simulink model "Khajuriwala_rishi_rbe_595_hw_08_simulink"  (R2017b)
settings: Solver=VariableStepAuto  StartTime=0.0  StopTime=10  RelTol=1e-3
values from neighbouring files (symbols this model uses):
  bc = bh    (= 25)    [Khajuriwala_rishi_rbe_595_hw_08_initialization_file.m]
  bh = 25    [Khajuriwala_rishi_rbe_595_hw_08_initialization_file.m]
  Bt = 300    [Khajuriwala_rishi_rbe_595_hw_08_initialization_file.m]    (also in virtualcoupling3.m = block.DialogPrm(2).Data)
  Bvc = 3    [Khajuriwala_rishi_rbe_595_hw_08_initialization_file.m]    (also in virtualcoupling1.m = block.DialogPrm(2).Data)
  Fh = 5    [Khajuriwala_rishi_rbe_595_hw_08_initialization_file.m]
  fh1 = 5    [Khajuriwala_rishi_rbe_595_hw_08_initialization_file.m]
  Kt = 2000    [Khajuriwala_rishi_rbe_595_hw_08_initialization_file.m]    (also in virtualcoupling3.m = block.DialogPrm(1).Data)
  Kvc = 2000    [Khajuriwala_rishi_rbe_595_hw_08_initialization_file.m]    (also in virtualcoupling1.m = block.DialogPrm(1).Data)
  mc = 20    [Khajuriwala_rishi_rbe_595_hw_08_initialization_file.m]
  mh = 10    [Khajuriwala_rishi_rbe_595_hw_08_initialization_file.m]
  vc0 = vhd0    (= 0)    [Khajuriwala_rishi_rbe_595_hw_08_initialization_file.m]
  vhd0 = 0    [Khajuriwala_rishi_rbe_595_hw_08_initialization_file.m]
  xc0 = xhd0    (= -0.05)    [Khajuriwala_rishi_rbe_595_hw_08_initialization_file.m]
  xhd0 = -0.05    [Khajuriwala_rishi_rbe_595_hw_08_initialization_file.m]
settings Model: Creator=Lhotse  LastModifiedBy=Lhotse

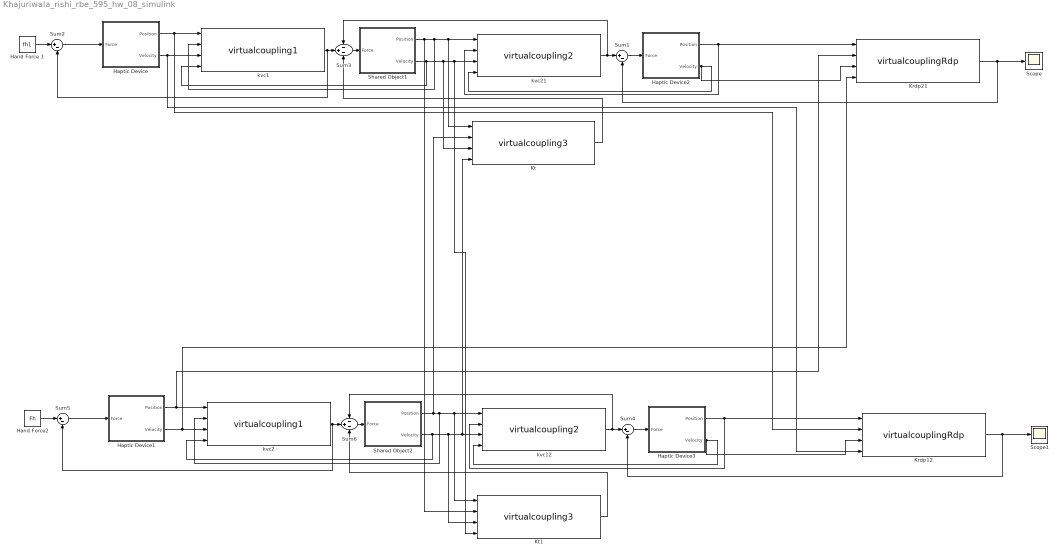
== system Khajuriwala_rishi_rbe_595_hw_08_simulink ==
  Hand Force 1 : Constant  Value=fh1
  Hand Force2 : Constant  Value=Fh
  Haptic Device : Subsystem
  Haptic Device1 : Subsystem
  Haptic Device2 : Subsystem
  Haptic Device3 : Subsystem
  Krdp12 : M-S-Function  FunctionName=virtualcouplingRdp  Parameters=Krdp, Brdp
  Krdp21 : M-S-Function  FunctionName=virtualcouplingRdp  Parameters=Krdp, Brdp
  Kt : M-S-Function  FunctionName=virtualcoupling3  Parameters=Kt,Bt
  Kt1 : M-S-Function  FunctionName=virtualcoupling3  Parameters=Kt,Bt
  Scope : Scope
  Scope1 : Scope
  Shared Object1 : Subsystem
  Shared Object2 : Subsystem
  Sum{1..2,4..5} (4 alike) : Sum  Inputs=|+-
  Sum3 : Sum  Inputs=-+-
  Sum6 : Sum  Inputs=-+-
  kvc1 : M-S-Function  FunctionName=virtualcoupling1  Parameters=Kvc,Bvc
  kvc12 : M-S-Function  FunctionName=virtualcoupling2  Parameters=Kvc,Bvc
  kvc2 : M-S-Function  FunctionName=virtualcoupling1  Parameters=Kvc,Bvc
  kvc21 : M-S-Function  FunctionName=virtualcoupling2  Parameters=Kvc,Bvc
  wires:
  Haptic Device/1(Position) -> Krdp12/2, kvc1/1
  Shared Object1/2(Velocity) -> Kt/3, Kt1/4, kvc21/3, kvc1/4
  Haptic Device2/2(Velocity) -> kvc21/4, Krdp21/3
  Haptic Device/2(Velocity) -> Krdp12/4, kvc1/3
  Shared Object1/1(Position) -> Kt1/2, Kt/1, kvc21/1, kvc1/2
  Sum2/1 -> Haptic Device/1(Force)
  Haptic Device2/1(Position) -> kvc21/2, Krdp21/1
  Hand Force 1/1 -> Sum2/1
  kvc21/1 -> Sum3/1, Sum1/1
  Sum1/1 -> Haptic Device2/1(Force)
  kvc1/1 -> Sum3/2, Sum2/2
  Sum3/1 -> Shared Object1/1(Force)
  Kt/1 -> Sum3/3
  Krdp21/1 -> Sum1/2, Scope/1
  kvc12/1 -> Sum6/1, Sum4/1
  Sum4/1 -> Haptic Device3/1(Force)
  kvc2/1 -> Sum6/2, Sum5/2
  Sum6/1 -> Shared Object2/1(Force)
  Hand Force2/1 -> Sum5/1
  Haptic Device1/2(Velocity) -> Krdp21/4, kvc2/3
  Haptic Device3/1(Position) -> kvc12/2, Krdp12/1
  Haptic Device3/2(Velocity) -> kvc12/4, Krdp12/3
  Sum5/1 -> Haptic Device1/1(Force)
  Haptic Device1/1(Position) -> Krdp21/2, kvc2/1
  Shared Object2/1(Position) -> Kt/2, Kt1/1, kvc12/1, kvc2/2
  Kt1/1 -> Sum6/3
  Krdp12/1 -> Sum4/2, Scope1/1
  Shared Object2/2(Velocity) -> Kt1/3, Kt/4, kvc12/3, kvc2/4

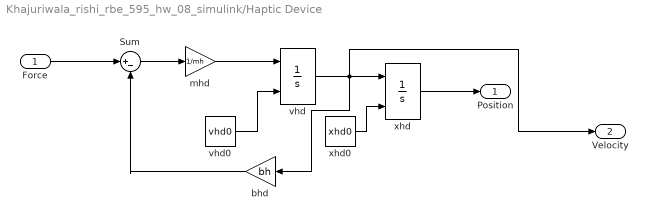
== system Khajuriwala_rishi_rbe_595_hw_08_simulink/Haptic Device ==
  Force : Inport
  Sum : Sum  Inputs=|+-
  bhd : Gain  Gain=bh
  mhd : Gain  Gain=1/mh
  vhd : Integrator  InitialConditionSource=external
  vhd0 : Constant  Value=vhd0
  xhd : Integrator  InitialConditionSource=external
  xhd0 : Constant  Value=xhd0
  Position : Outport
  Velocity : Outport  Port=2
  wires:
  vhd0/1 -> vhd/2
  xhd0/1 -> xhd/2
  mhd/1 -> vhd/1
  Force/1 -> Sum/1
  xhd/1 -> Position/1
  bhd/1 -> Sum/2
  vhd/1 -> bhd/1, Velocity/1, xhd/1
  Sum/1 -> mhd/1

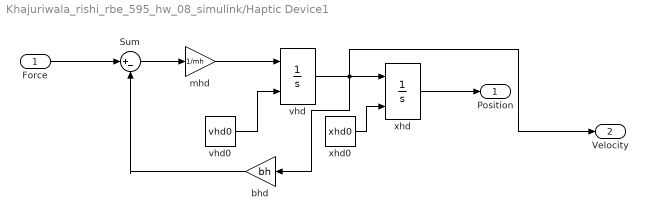
== system Khajuriwala_rishi_rbe_595_hw_08_simulink/Haptic Device1 ==
  Force : Inport
  Sum : Sum  Inputs=|+-
  bhd : Gain  Gain=bh
  mhd : Gain  Gain=1/mh
  vhd : Integrator  InitialConditionSource=external
  vhd0 : Constant  Value=vhd0
  xhd : Integrator  InitialConditionSource=external
  xhd0 : Constant  Value=xhd0
  Position : Outport
  Velocity : Outport  Port=2
  wires:
  vhd0/1 -> vhd/2
  xhd0/1 -> xhd/2
  mhd/1 -> vhd/1
  Force/1 -> Sum/1
  xhd/1 -> Position/1
  bhd/1 -> Sum/2
  vhd/1 -> bhd/1, Velocity/1, xhd/1
  Sum/1 -> mhd/1

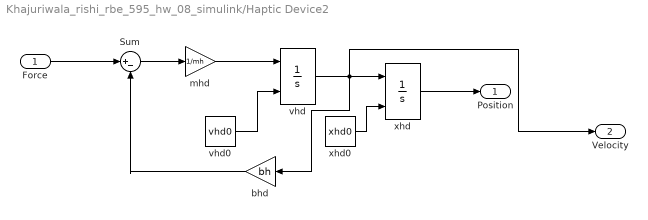
== system Khajuriwala_rishi_rbe_595_hw_08_simulink/Haptic Device2 ==
  Force : Inport
  Sum : Sum  Inputs=|+-
  bhd : Gain  Gain=bh
  mhd : Gain  Gain=1/mh
  vhd : Integrator  InitialConditionSource=external
  vhd0 : Constant  Value=vhd0
  xhd : Integrator  InitialConditionSource=external
  xhd0 : Constant  Value=xhd0
  Position : Outport
  Velocity : Outport  Port=2
  wires:
  vhd0/1 -> vhd/2
  xhd0/1 -> xhd/2
  mhd/1 -> vhd/1
  Force/1 -> Sum/1
  xhd/1 -> Position/1
  bhd/1 -> Sum/2
  vhd/1 -> bhd/1, Velocity/1, xhd/1
  Sum/1 -> mhd/1

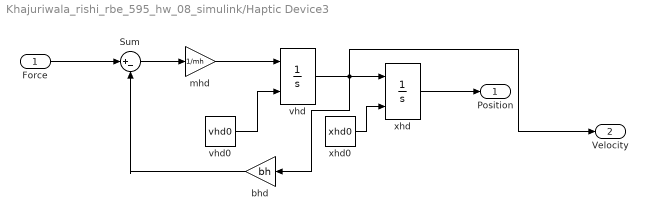
== system Khajuriwala_rishi_rbe_595_hw_08_simulink/Haptic Device3 ==
  Force : Inport
  Sum : Sum  Inputs=|+-
  bhd : Gain  Gain=bh
  mhd : Gain  Gain=1/mh
  vhd : Integrator  InitialConditionSource=external
  vhd0 : Constant  Value=vhd0
  xhd : Integrator  InitialConditionSource=external
  xhd0 : Constant  Value=xhd0
  Position : Outport
  Velocity : Outport  Port=2
  wires:
  vhd0/1 -> vhd/2
  xhd0/1 -> xhd/2
  mhd/1 -> vhd/1
  Force/1 -> Sum/1
  xhd/1 -> Position/1
  bhd/1 -> Sum/2
  vhd/1 -> bhd/1, Velocity/1, xhd/1
  Sum/1 -> mhd/1

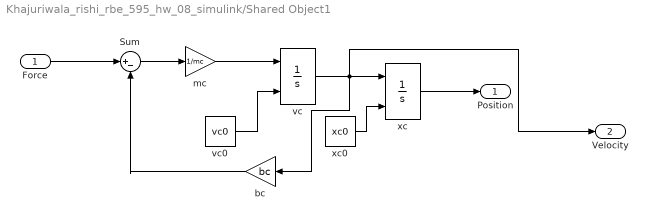
== system Khajuriwala_rishi_rbe_595_hw_08_simulink/Shared Object1 ==
  Force : Inport
  Sum : Sum  Inputs=|+-
  "bc " : Gain  Gain=bc
  mc : Gain  Gain=1/mc
  vc : Integrator  InitialConditionSource=external
  vc0 : Constant  Value=vc0
  xc : Integrator  InitialConditionSource=external
  xc0 : Constant  Value=xc0
  Position : Outport
  Velocity : Outport  Port=2
  wires:
  vc0/1 -> vc/2
  xc0/1 -> xc/2
  mc/1 -> vc/1
  Force/1 -> Sum/1
  xc/1 -> Position/1
  "bc "/1 -> Sum/2
  vc/1 -> "bc "/1, Velocity/1, xc/1
  Sum/1 -> mc/1

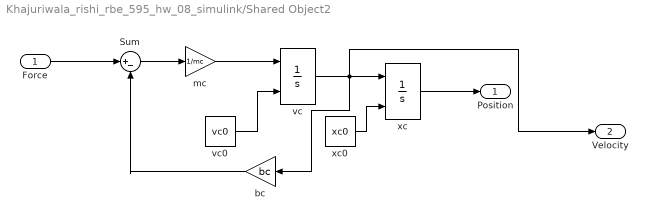
== system Khajuriwala_rishi_rbe_595_hw_08_simulink/Shared Object2 ==
  Force : Inport
  Sum : Sum  Inputs=|+-
  "bc " : Gain  Gain=bc
  mc : Gain  Gain=1/mc
  vc : Integrator  InitialConditionSource=external
  vc0 : Constant  Value=vc0
  xc : Integrator  InitialConditionSource=external
  xc0 : Constant  Value=xc0
  Position : Outport
  Velocity : Outport  Port=2
  wires:
  vc0/1 -> vc/2
  xc0/1 -> xc/2
  mc/1 -> vc/1
  Force/1 -> Sum/1
  xc/1 -> Position/1
  "bc "/1 -> Sum/2
  vc/1 -> "bc "/1, Velocity/1, xc/1
  Sum/1 -> mc/1
